simulink model "simu_21a"  (R2021a)
settings: Solver=VariableStepAuto  StartTime=0.0  StopTime=6  RelTol=1e-3
settings Model: Creator=admin  LastModifiedBy=psp_dada
settings ConfigComp: CovBoundaryAbsTol=1.0e-5

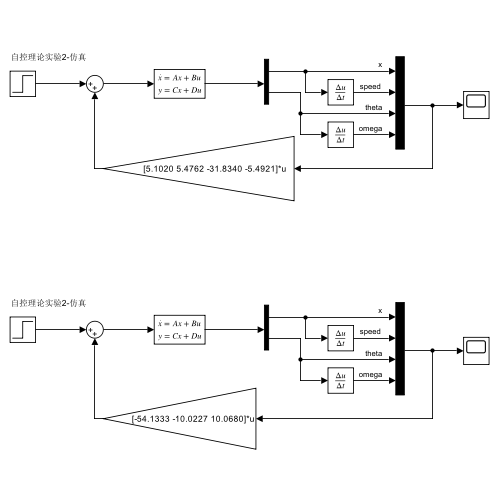
[thumbnail: Simulink's stored preview of the top-level diagram]
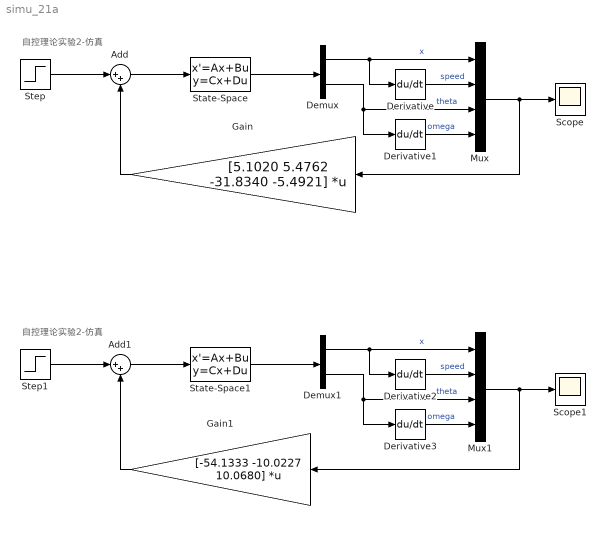
== system simu_21a ==
  note: 自控理论实验2-仿真
  note: 自控理论实验2-仿真
  Add : Sum  Inputs=|++
  Add1 : Sum  Inputs=|++
  Demux : Demux  Outputs=2
  Demux1 : Demux  Outputs=2
  Derivative{,1..3} (4 alike) : Derivative
  Gain : Gain  Gain=[5.1020 5.4762 -31.8340 -5.4921]  Multiplication=Matrix(K*u)
  Gain1 : Gain  Gain=[-54.1333 -10.0227 10.0680]  Multiplication=Matrix(K*u)
  Mux : Mux
  Mux1 : Mux
  Scope : Scope
  Scope1 : Scope
  State-Space : StateSpace  A=[0 1 0 0;0 0 0 0;0 0 0 1;0 0 29.4 0]  B=[0;1;0;3]  C=[1 0 0 0;0 0 1 0]  D=[0;0]  InitialCondition=0
  State-Space1 : StateSpace  A=[0 1 0;29.4 0 0; 0 0 0]  B=[0; 3; 1]  C=[1 0 0]  D=[0]  InitialCondition=0
  Step : Step  Time=0.5  SampleTime=0
  Step1 : Step  Time=0.5  SampleTime=0
  wires:
  Gain/1 -> Add/2
  Add/1 -> State-Space/1
  State-Space/1 -> Demux/1
  Step/1 -> Add/1
  Demux/1 -> Mux/1, Derivative/1  "x"
  Mux/1 -> Gain/1, Scope/1
  Derivative/1 -> Mux/2  "speed"
  Demux/2 -> Derivative1/1, Mux/3  "theta"
  Derivative1/1 -> Mux/4  "omega"
  Mux1/1 -> Gain1/1, Scope1/1
  Demux1/1 -> Mux1/1, Derivative2/1  "x"
  Gain1/1 -> Add1/2
  Step1/1 -> Add1/1
  Derivative2/1 -> Mux1/2  "speed"
  Derivative3/1 -> Mux1/4  "omega"
  State-Space1/1 -> Demux1/1
  Add1/1 -> State-Space1/1
  Demux1/2 -> Derivative3/1, Mux1/3  "theta"
